simulink model "HybridBus_BackwardModel_pre_supervisory_refactor"  (R2025a)
settings: Solver=FixedStepDiscrete  StartTime=0.0  StopTime=model_stop_time_s  FixedStep=model_sample_time_s  RelTol=1e-3
InitFcn:
  | assign_hybrid_bus_model_workspace;
undefined symbols (not defined in the file or in its folder): air_density_kg_m3, auxiliary_base_power_kw, auxiliary_override, battery1_charge_efficiency, battery1_discharge_efficiency, battery1_initial_energy_kwh, battery1_max_charge_kw, battery1_max_discharge_kw, battery1_max_energy_kwh, battery1_max_soe, battery1_min_energy_kwh, battery1_usable_energy_kwh, battery2_charge_efficiency, battery2_discharge_efficiency, battery2_initial_energy_kwh, battery2_max_charge_kw, battery2_max_discharge_kw, battery2_max_energy_kwh, battery2_max_soe, battery2_min_energy_kwh, battery2_usable_energy_kwh, battery_full_detection_margin, battery_role_switch_soe, DiscIntNeverNeededParam, drag_coefficient, electricity_price_per_kWh, final_drive_motoring_efficiency, final_drive_ratio, final_drive_regen_efficiency, frontal_area_m2, fuel_price_per_L, genset_charge_target_soe, genset_fuel_L_per_kWh, genset_max_power_kw, genset_optimum_power_kw, gravity_m_s2, grid_charge_efficiency, initial_active_battery_is_1, model_sample_time_s, motor_max_speed_rpm, motor_motoring_efficiency, motor_regen_efficiency, motor_regen_limit_kw, motor_traction_limit_kw, rolling_coefficient, tyre_radius_m, vehicle_mass_kg
settings Model: Creator=Karuna  LastModifiedBy=Karuna
settings DataIOCC: SaveOutput=off  SignalLogging=off

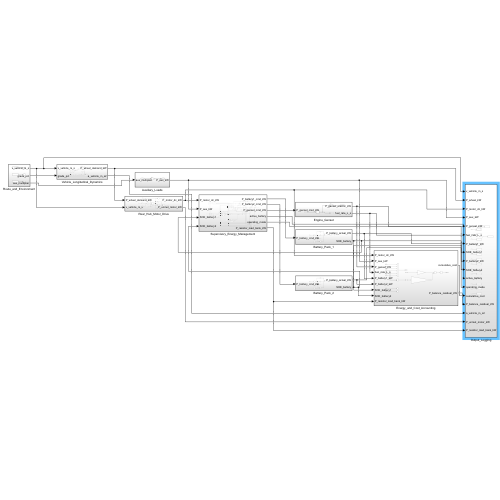
[thumbnail: Simulink's stored preview of the top-level diagram]
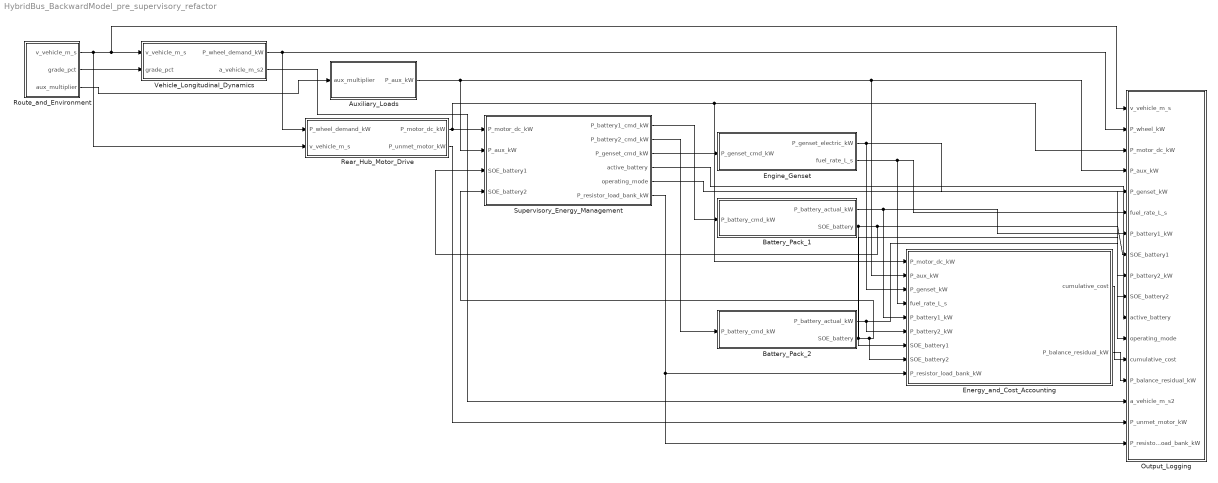
== system HybridBus_BackwardModel_pre_supervisory_refactor ==
  Auxiliary_Loads : Subsystem
  Battery_Pack_1 : Subsystem
  Battery_Pack_2 : Subsystem
  Energy_and_Cost_Accounting : Subsystem
  Engine_Genset : Subsystem
  Output_Logging : Subsystem
  Rear_Hub_Motor_Drive : Subsystem
  Route_and_Environment : Subsystem
  Supervisory_Energy_Management : Subsystem
  Vehicle_Longitudinal_Dynamics : Subsystem
  wires:
  Battery_Pack_2/2(SOE_battery) -> Supervisory_Energy_Management/4(SOE_battery2), Energy_and_Cost_Accounting/8(SOE_battery2), Output_Logging/10(SOE_battery2)
  Route_and_Environment/3(aux_multiplier) -> Auxiliary_Loads/1(aux_multiplier)
  Route_and_Environment/2(grade_pct) -> Vehicle_Longitudinal_Dynamics/2(grade_pct)
  Route_and_Environment/1(v_vehicle_m_s) -> Output_Logging/1(v_vehicle_m_s), Vehicle_Longitudinal_Dynamics/1(v_vehicle_m_s), Rear_Hub_Motor_Drive/2(v_vehicle_m_s)
  Vehicle_Longitudinal_Dynamics/1(P_wheel_demand_kW) -> Output_Logging/2(P_wheel_kW), Rear_Hub_Motor_Drive/1(P_wheel_demand_kW)
  Vehicle_Longitudinal_Dynamics/2(a_vehicle_m_s2) -> Output_Logging/15(a_vehicle_m_s2)
  Auxiliary_Loads/1(P_aux_kW) -> Energy_and_Cost_Accounting/2(P_aux_kW), Output_Logging/4(P_aux_kW), Supervisory_Energy_Management/2(P_aux_kW)
  Rear_Hub_Motor_Drive/2(P_unmet_motor_kW) -> Output_Logging/16(P_unmet_motor_kW)
  Rear_Hub_Motor_Drive/1(P_motor_dc_kW) -> Energy_and_Cost_Accounting/1(P_motor_dc_kW), Output_Logging/3(P_motor_dc_kW), Supervisory_Energy_Management/1(P_motor_dc_kW)
  Engine_Genset/2(fuel_rate_L_s) -> Energy_and_Cost_Accounting/4(fuel_rate_L_s), Output_Logging/6(fuel_rate_L_s)
  Supervisory_Energy_Management/1(P_battery1_cmd_kW) -> Battery_Pack_1/1(P_battery_cmd_kW)
  Supervisory_Energy_Management/2(P_battery2_cmd_kW) -> Battery_Pack_2/1(P_battery_cmd_kW)
  Engine_Genset/1(P_genset_electric_kW) -> Output_Logging/5(P_genset_kW), Energy_and_Cost_Accounting/3(P_genset_kW)
  Supervisory_Energy_Management/3(P_genset_cmd_kW) -> Engine_Genset/1(P_genset_cmd_kW)
  Supervisory_Energy_Management/4(active_battery) -> Output_Logging/11(active_battery)
  Supervisory_Energy_Management/5(operating_mode) -> Output_Logging/12(operating_mode)
  Supervisory_Energy_Management/6(P_resistor_load_bank_kW) -> Energy_and_Cost_Accounting/9(P_resistor_load_bank_kW), Output_Logging/17(P_resistor_load_bank_kW)
  Battery_Pack_1/1(P_battery_actual_kW) -> Output_Logging/7(P_battery1_kW), Energy_and_Cost_Accounting/5(P_battery1_kW)
  Battery_Pack_1/2(SOE_battery) -> Supervisory_Energy_Management/3(SOE_battery1), Output_Logging/8(SOE_battery1), Energy_and_Cost_Accounting/7(SOE_battery1)
  Battery_Pack_2/1(P_battery_actual_kW) -> Output_Logging/9(P_battery2_kW), Energy_and_Cost_Accounting/6(P_battery2_kW)
  Energy_and_Cost_Accounting/1(cumulative_cost) -> Output_Logging/13(cumulative_cost)
  Energy_and_Cost_Accounting/2(P_balance_residual_kW) -> Output_Logging/14(P_balance_residual_kW)

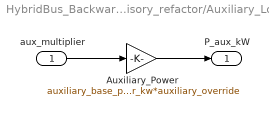
== system HybridBus_BackwardModel_pre_supervisory_refactor/Auxiliary_Loads ==
  aux_multiplier : Inport
  Auxiliary_Power : Gain  Gain=auxiliary_base_power_kw*auxiliary_override
  P_aux_kW : Outport
  wires:
  Auxiliary_Power/1 -> P_aux_kW/1
  aux_multiplier/1 -> Auxiliary_Power/1

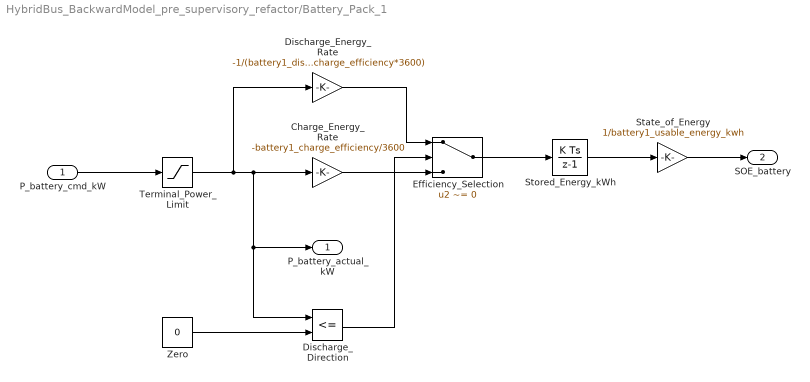
== system HybridBus_BackwardModel_pre_supervisory_refactor/Battery_Pack_1 ==
  P_battery_cmd_kW : Inport
  Charge_Energy_Rate : Gain  Gain=-battery1_charge_efficiency/3600
  Discharge_Direction : RelationalOperator  Operator=<=  OutDataTypeStr=boolean  RndMeth=Simplest  InputSameDT=off
  Discharge_Energy_Rate : Gain  Gain=-1/(battery1_discharge_efficiency*3600)
  Efficiency_Selection : Switch  Criteria=u2 ~= 0  SaturateOnIntegerOverflow=off  InputSameDT=off
  State_of_Energy : Gain  Gain=1/battery1_usable_energy_kwh
  Stored_Energy_kWh : DiscreteIntegrator  InitialCondition=battery1_initial_energy_kwh  SampleTime=model_sample_time_s  LimitOutput=on  UpperSaturationLimit=battery1_max_energy_kwh  LowerSaturationLimit=battery1_min_energy_kwh  ICPrevOutput=DiscIntNeverNeededParam  ICPrevScaledInput=DiscIntNeverNeededParam
  Terminal_Power_Limit : Saturate  UpperLimit=battery1_max_discharge_kw  LowerLimit=-battery1_max_charge_kw
  Zero : Constant  Value=0
  P_battery_actual_kW : Outport
  SOE_battery : Outport  Port=2
  wires:
  State_of_Energy/1 -> SOE_battery/1
  Stored_Energy_kWh/1 -> State_of_Energy/1
  Efficiency_Selection/1 -> Stored_Energy_kWh/1
  Charge_Energy_Rate/1 -> Efficiency_Selection/3
  Discharge_Direction/1 -> Efficiency_Selection/2
  Discharge_Energy_Rate/1 -> Efficiency_Selection/1
  Zero/1 -> Discharge_Direction/2
  Terminal_Power_Limit/1 -> P_battery_actual_kW/1, Discharge_Direction/1, Charge_Energy_Rate/1, Discharge_Energy_Rate/1
  P_battery_cmd_kW/1 -> Terminal_Power_Limit/1

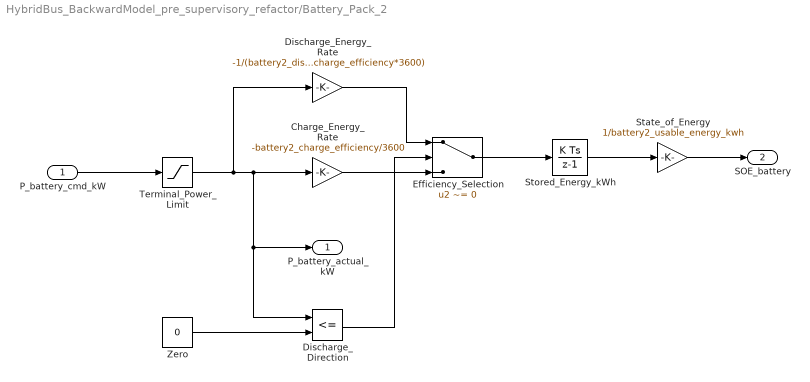
== system HybridBus_BackwardModel_pre_supervisory_refactor/Battery_Pack_2 ==
  P_battery_cmd_kW : Inport
  Charge_Energy_Rate : Gain  Gain=-battery2_charge_efficiency/3600
  Discharge_Direction : RelationalOperator  Operator=<=  OutDataTypeStr=boolean  RndMeth=Simplest  InputSameDT=off
  Discharge_Energy_Rate : Gain  Gain=-1/(battery2_discharge_efficiency*3600)
  Efficiency_Selection : Switch  Criteria=u2 ~= 0  SaturateOnIntegerOverflow=off  InputSameDT=off
  State_of_Energy : Gain  Gain=1/battery2_usable_energy_kwh
  Stored_Energy_kWh : DiscreteIntegrator  InitialCondition=battery2_initial_energy_kwh  SampleTime=model_sample_time_s  LimitOutput=on  UpperSaturationLimit=battery2_max_energy_kwh  LowerSaturationLimit=battery2_min_energy_kwh  ICPrevOutput=DiscIntNeverNeededParam  ICPrevScaledInput=DiscIntNeverNeededParam
  Terminal_Power_Limit : Saturate  UpperLimit=battery2_max_discharge_kw  LowerLimit=-battery2_max_charge_kw
  Zero : Constant  Value=0
  P_battery_actual_kW : Outport
  SOE_battery : Outport  Port=2
  wires:
  State_of_Energy/1 -> SOE_battery/1
  Stored_Energy_kWh/1 -> State_of_Energy/1
  Efficiency_Selection/1 -> Stored_Energy_kWh/1
  Charge_Energy_Rate/1 -> Efficiency_Selection/3
  Discharge_Direction/1 -> Efficiency_Selection/2
  Discharge_Energy_Rate/1 -> Efficiency_Selection/1
  Zero/1 -> Discharge_Direction/2
  Terminal_Power_Limit/1 -> P_battery_actual_kW/1, Discharge_Direction/1, Charge_Energy_Rate/1, Discharge_Energy_Rate/1
  P_battery_cmd_kW/1 -> Terminal_Power_Limit/1

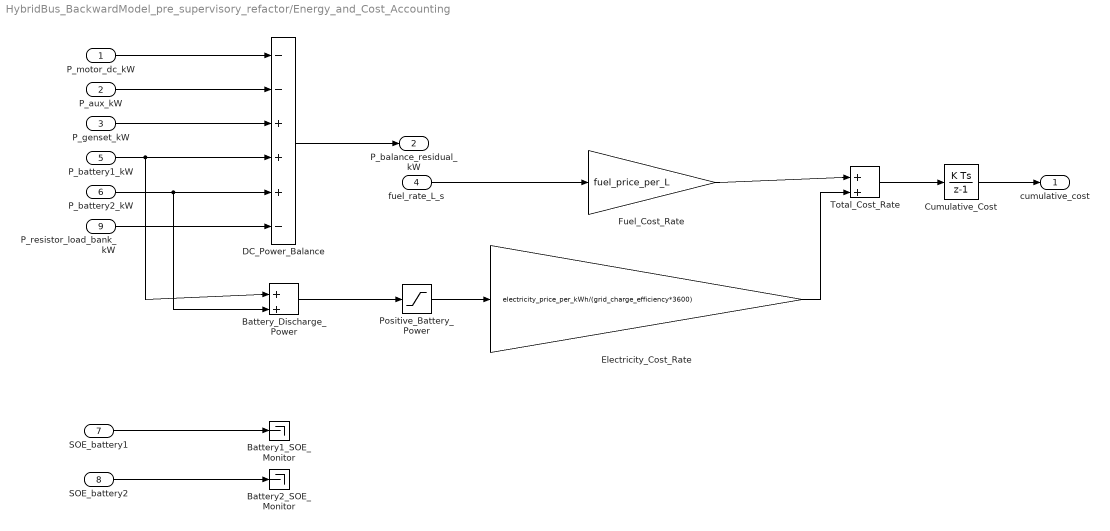
== system HybridBus_BackwardModel_pre_supervisory_refactor/Energy_and_Cost_Accounting ==
  P_motor_dc_kW : Inport
  P_aux_kW : Inport  Port=2
  P_genset_kW : Inport  Port=3
  fuel_rate_L_s : Inport  Port=4
  P_battery1_kW : Inport  Port=5
  P_battery2_kW : Inport  Port=6
  SOE_battery1 : Inport  Port=7
  SOE_battery2 : Inport  Port=8
  P_resistor_load_bank_kW : Inport  Port=9
  Battery1_SOE_Monitor : Terminator
  Battery2_SOE_Monitor : Terminator
  Battery_Discharge_Power : Sum  Inputs=|++
  Cumulative_Cost : DiscreteIntegrator  SampleTime=model_sample_time_s  ICPrevOutput=DiscIntNeverNeededParam  ICPrevScaledInput=DiscIntNeverNeededParam
  DC_Power_Balance : Sum  Inputs=--+++-
  Electricity_Cost_Rate : Gain  Gain=electricity_price_per_kWh/(grid_charge_efficiency*3600)
  Fuel_Cost_Rate : Gain  Gain=fuel_price_per_L
  Positive_Battery_Power : Saturate  UpperLimit=inf  LowerLimit=0
  Total_Cost_Rate : Sum  Inputs=|++
  cumulative_cost : Outport
  P_balance_residual_kW : Outport  Port=2
  wires:
  fuel_rate_L_s/1 -> Fuel_Cost_Rate/1
  P_aux_kW/1 -> DC_Power_Balance/2
  P_battery2_kW/1 -> Battery_Discharge_Power/2, DC_Power_Balance/5
  P_motor_dc_kW/1 -> DC_Power_Balance/1
  P_genset_kW/1 -> DC_Power_Balance/3
  P_battery1_kW/1 -> Battery_Discharge_Power/1, DC_Power_Balance/4
  SOE_battery2/1 -> Battery2_SOE_Monitor/1
  Battery_Discharge_Power/1 -> Positive_Battery_Power/1
  P_resistor_load_bank_kW/1 -> DC_Power_Balance/6
  SOE_battery1/1 -> Battery1_SOE_Monitor/1
  Cumulative_Cost/1 -> cumulative_cost/1
  DC_Power_Balance/1 -> P_balance_residual_kW/1
  Total_Cost_Rate/1 -> Cumulative_Cost/1
  Positive_Battery_Power/1 -> Electricity_Cost_Rate/1
  Fuel_Cost_Rate/1 -> Total_Cost_Rate/1
  Electricity_Cost_Rate/1 -> Total_Cost_Rate/2

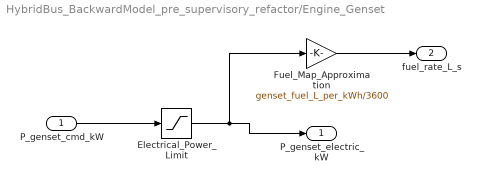
== system HybridBus_BackwardModel_pre_supervisory_refactor/Engine_Genset ==
  P_genset_cmd_kW : Inport
  Electrical_Power_Limit : Saturate  UpperLimit=genset_max_power_kw  LowerLimit=0
  Fuel_Map_Approximation : Gain  Gain=genset_fuel_L_per_kWh/3600
  P_genset_electric_kW : Outport
  fuel_rate_L_s : Outport  Port=2
  wires:
  Fuel_Map_Approximation/1 -> fuel_rate_L_s/1
  Electrical_Power_Limit/1 -> P_genset_electric_kW/1, Fuel_Map_Approximation/1
  P_genset_cmd_kW/1 -> Electrical_Power_Limit/1

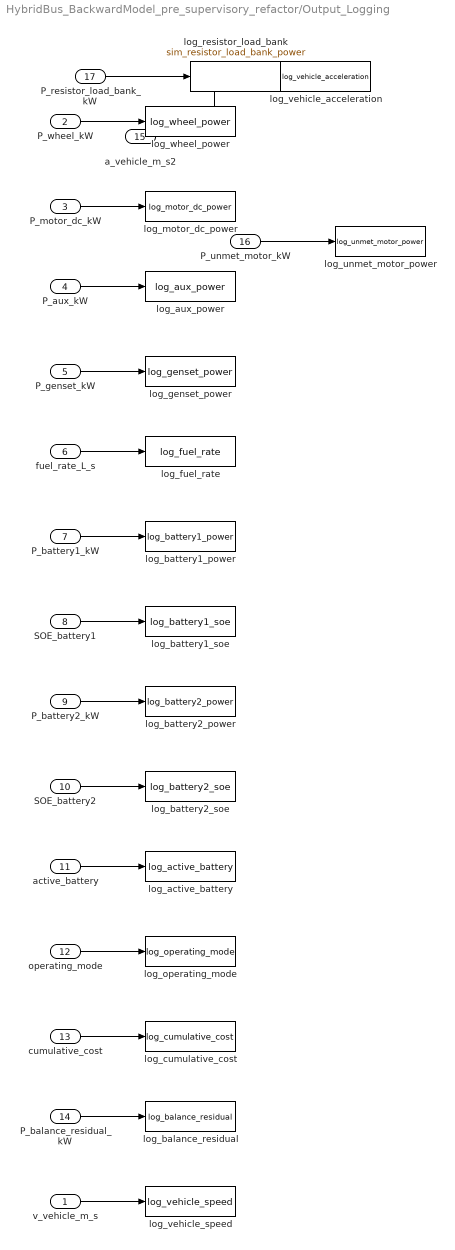
== system HybridBus_BackwardModel_pre_supervisory_refactor/Output_Logging ==
  v_vehicle_m_s : Inport
  P_wheel_kW : Inport  Port=2
  P_motor_dc_kW : Inport  Port=3
  P_aux_kW : Inport  Port=4
  P_genset_kW : Inport  Port=5
  fuel_rate_L_s : Inport  Port=6
  P_battery1_kW : Inport  Port=7
  SOE_battery1 : Inport  Port=8
  P_battery2_kW : Inport  Port=9
  SOE_battery2 : Inport  Port=10
  active_battery : Inport  Port=11
  operating_mode : Inport  Port=12
  cumulative_cost : Inport  Port=13
  P_balance_residual_kW : Inport  Port=14
  a_vehicle_m_s2 : Inport  Port=15
  P_unmet_motor_kW : Inport  Port=16
  P_resistor_load_bank_kW : Inport  Port=17
  log_active_battery : ToWorkspace  VariableName=log_active_battery  SaveFormat=Timeseries  SampleTime=-1
  log_aux_power : ToWorkspace  VariableName=log_aux_power  SaveFormat=Timeseries  SampleTime=-1
  log_balance_residual : ToWorkspace  VariableName=log_balance_residual  SaveFormat=Timeseries  SampleTime=-1
  log_battery1_power : ToWorkspace  VariableName=log_battery1_power  SaveFormat=Timeseries  SampleTime=-1
  log_battery1_soe : ToWorkspace  VariableName=log_battery1_soe  SaveFormat=Timeseries  SampleTime=-1
  log_battery2_power : ToWorkspace  VariableName=log_battery2_power  SaveFormat=Timeseries  SampleTime=-1
  log_battery2_soe : ToWorkspace  VariableName=log_battery2_soe  SaveFormat=Timeseries  SampleTime=-1
  log_cumulative_cost : ToWorkspace  VariableName=log_cumulative_cost  SaveFormat=Timeseries  SampleTime=-1
  log_fuel_rate : ToWorkspace  VariableName=log_fuel_rate  SaveFormat=Timeseries  SampleTime=-1
  log_genset_power : ToWorkspace  VariableName=log_genset_power  SaveFormat=Timeseries  SampleTime=-1
  log_motor_dc_power : ToWorkspace  VariableName=log_motor_dc_power  SaveFormat=Timeseries  SampleTime=-1
  log_operating_mode : ToWorkspace  VariableName=log_operating_mode  SaveFormat=Timeseries  SampleTime=-1
  log_resistor_load_bank : ToWorkspace  VariableName=sim_resistor_load_bank_power  SampleTime=-1
  log_unmet_motor_power : ToWorkspace  VariableName=log_unmet_motor_power  SaveFormat=Timeseries  SampleTime=-1
  log_vehicle_acceleration : ToWorkspace  VariableName=log_vehicle_acceleration  SaveFormat=Timeseries  SampleTime=-1
  log_vehicle_speed : ToWorkspace  VariableName=log_vehicle_speed  SaveFormat=Timeseries  SampleTime=-1
  log_wheel_power : ToWorkspace  VariableName=log_wheel_power  SaveFormat=Timeseries  SampleTime=-1
  wires:
  P_balance_residual_kW/1 -> log_balance_residual/1
  cumulative_cost/1 -> log_cumulative_cost/1
  operating_mode/1 -> log_operating_mode/1
  active_battery/1 -> log_active_battery/1
  SOE_battery2/1 -> log_battery2_soe/1
  P_battery2_kW/1 -> log_battery2_power/1
  SOE_battery1/1 -> log_battery1_soe/1
  P_battery1_kW/1 -> log_battery1_power/1
  fuel_rate_L_s/1 -> log_fuel_rate/1
  P_genset_kW/1 -> log_genset_power/1
  P_aux_kW/1 -> log_aux_power/1
  P_motor_dc_kW/1 -> log_motor_dc_power/1
  P_wheel_kW/1 -> log_wheel_power/1
  v_vehicle_m_s/1 -> log_vehicle_speed/1
  P_unmet_motor_kW/1 -> log_unmet_motor_power/1
  P_resistor_load_bank_kW/1 -> log_resistor_load_bank/1
  a_vehicle_m_s2/1 -> log_vehicle_acceleration/1

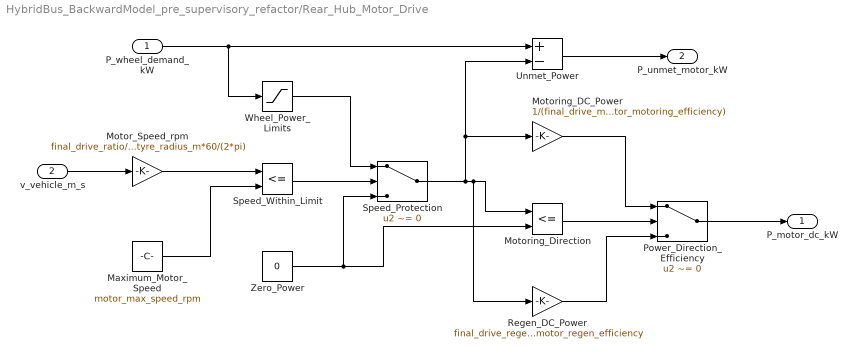
== system HybridBus_BackwardModel_pre_supervisory_refactor/Rear_Hub_Motor_Drive ==
  P_wheel_demand_kW : Inport
  v_vehicle_m_s : Inport  Port=2
  Maximum_Motor_Speed : Constant  Value=motor_max_speed_rpm
  Motor_Speed_rpm : Gain  Gain=final_drive_ratio/tyre_radius_m*60/(2*pi)
  Motoring_DC_Power : Gain  Gain=1/(final_drive_motoring_efficiency*motor_motoring_efficiency)
  Motoring_Direction : RelationalOperator  Operator=<=  OutDataTypeStr=boolean  RndMeth=Simplest  InputSameDT=off
  Power_Direction_Efficiency : Switch  Criteria=u2 ~= 0  SaturateOnIntegerOverflow=off  InputSameDT=off
  Regen_DC_Power : Gain  Gain=final_drive_regen_efficiency*motor_regen_efficiency
  Speed_Protection : Switch  Criteria=u2 ~= 0  SaturateOnIntegerOverflow=off  InputSameDT=off
  Speed_Within_Limit : RelationalOperator  Operator=<=  OutDataTypeStr=boolean  RndMeth=Simplest  InputSameDT=off
  Unmet_Power : Sum  Inputs=+-
  Wheel_Power_Limits : Saturate  UpperLimit=motor_traction_limit_kw  LowerLimit=-motor_regen_limit_kw
  Zero_Power : Constant  Value=0
  P_motor_dc_kW : Outport
  P_unmet_motor_kW : Outport  Port=2
  wires:
  Unmet_Power/1 -> P_unmet_motor_kW/1
  Power_Direction_Efficiency/1 -> P_motor_dc_kW/1
  Regen_DC_Power/1 -> Power_Direction_Efficiency/3
  Motoring_Direction/1 -> Power_Direction_Efficiency/2
  Motoring_DC_Power/1 -> Power_Direction_Efficiency/1
  Speed_Protection/1 -> Regen_DC_Power/1, Motoring_Direction/1, Motoring_DC_Power/1, Unmet_Power/2
  Zero_Power/1 -> Speed_Protection/3, Motoring_Direction/2
  Speed_Within_Limit/1 -> Speed_Protection/2
  Wheel_Power_Limits/1 -> Speed_Protection/1
  Maximum_Motor_Speed/1 -> Speed_Within_Limit/2
  Motor_Speed_rpm/1 -> Speed_Within_Limit/1
  v_vehicle_m_s/1 -> Motor_Speed_rpm/1
  P_wheel_demand_kW/1 -> Unmet_Power/1, Wheel_Power_Limits/1

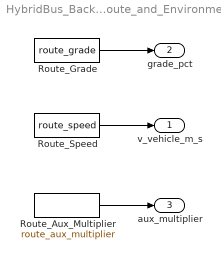
== system HybridBus_BackwardModel_pre_supervisory_refactor/Route_and_Environment ==
  Route_Aux_Multiplier : FromWorkspace  VariableName=route_aux_multiplier
  Route_Grade : FromWorkspace  VariableName=route_grade
  Route_Speed : FromWorkspace  VariableName=route_speed
  v_vehicle_m_s : Outport
  grade_pct : Outport  Port=2
  aux_multiplier : Outport  Port=3
  wires:
  Route_Aux_Multiplier/1 -> aux_multiplier/1
  Route_Grade/1 -> grade_pct/1
  Route_Speed/1 -> v_vehicle_m_s/1

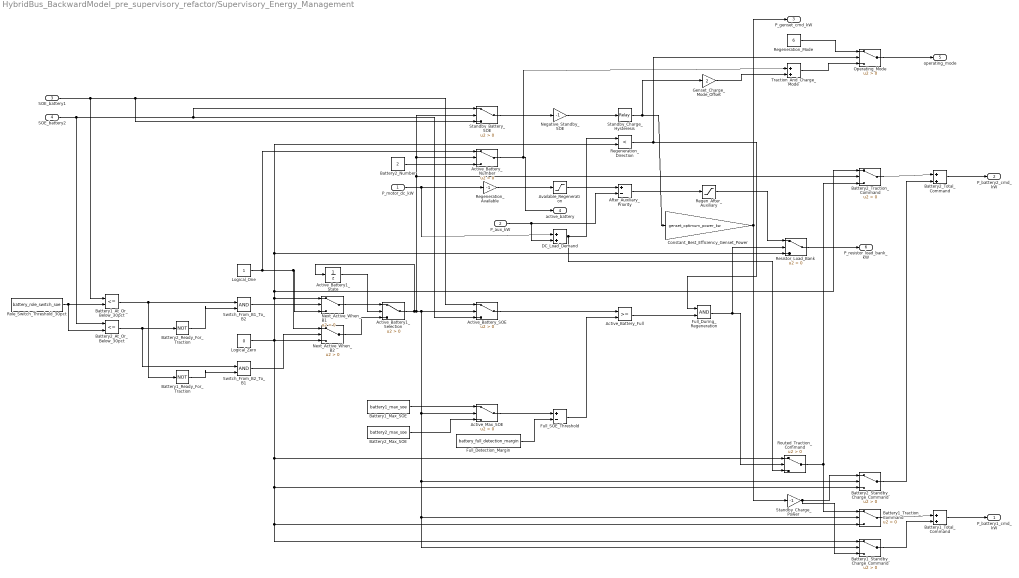
== system HybridBus_BackwardModel_pre_supervisory_refactor/Supervisory_Energy_Management ==
  P_motor_dc_kW : Inport
  P_aux_kW : Inport  Port=2
  SOE_battery1 : Inport  Port=3
  SOE_battery2 : Inport  Port=4
  Active_Battery1_Selection : Switch  Criteria=u2 > Threshold  SaturateOnIntegerOverflow=off  InputSameDT=off
  Active_Battery1_State : UnitDelay  InitialCondition=initial_active_battery_is_1  SampleTime=model_sample_time_s  HasFrameUpgradeWarning=on
  Active_Battery_Full : RelationalOperator  OutDataTypeStr=boolean  RndMeth=Simplest  InputSameDT=off
  Active_Battery_Number : Switch  Criteria=u2 > Threshold  SaturateOnIntegerOverflow=off  InputSameDT=off
  Active_Battery_SOE : Switch  Criteria=u2 > Threshold  SaturateOnIntegerOverflow=off  InputSameDT=off
  Active_Max_SOE : Switch  Criteria=u2 > Threshold  SaturateOnIntegerOverflow=off  InputSameDT=off
  After_Auxiliary_Priority : Sum  Inputs=+-
  Available_Regeneration : Saturate  UpperLimit=inf  LowerLimit=0
  Battery1_At_Or_Below_30pct : RelationalOperator  Operator=<=  OutDataTypeStr=boolean  RndMeth=Simplest  InputSameDT=off
  Battery1_Max_SOE : Constant  Value=battery1_max_soe
  Battery1_Ready_For_Traction : Logic  Operator=NOT  IconShape=distinctive  AllPortsSameDT=off  OutDataTypeStr=boolean
  Battery1_Standby_Charge_Command : Switch  Criteria=u2 > Threshold  SaturateOnIntegerOverflow=off  InputSameDT=off
  Battery1_Total_Command : Sum  Inputs=|++
  Battery1_Traction_Command : Switch  Criteria=u2 > Threshold  SaturateOnIntegerOverflow=off  InputSameDT=off
  Battery2_At_Or_Below_30pct : RelationalOperator  Operator=<=  OutDataTypeStr=boolean  RndMeth=Simplest  InputSameDT=off
  Battery2_Max_SOE : Constant  Value=battery2_max_soe
  Battery2_Number : Constant  Value=2
  Battery2_Ready_For_Traction : Logic  Operator=NOT  IconShape=distinctive  AllPortsSameDT=off  OutDataTypeStr=boolean
  Battery2_Standby_Charge_Command : Switch  Criteria=u2 > Threshold  SaturateOnIntegerOverflow=off  InputSameDT=off
  Battery2_Total_Command : Sum  Inputs=|++
  Battery2_Traction_Command : Switch  Criteria=u2 > Threshold  SaturateOnIntegerOverflow=off  InputSameDT=off
  Constant_Best_Efficiency_Genset_Power : Gain  Gain=genset_optimum_power_kw
  DC_Load_Demand : Sum  Inputs=|++
  Full_Detection_Margin : Constant  Value=battery_full_detection_margin
  Full_During_Regeneration : Logic  AllPortsSameDT=off  OutDataTypeStr=boolean
  Full_SOE_Threshold : Sum  Inputs=+-
  Genset_Charge_Mode_Offset : Gain  Gain=2
  Logical_One : Constant
  Logical_Zero : Constant  Value=0
  Negative_Standby_SOE : Gain  Gain=-1
  Next_Active_When_B1 : Switch  Criteria=u2 > Threshold  SaturateOnIntegerOverflow=off  InputSameDT=off
  Next_Active_When_B2 : Switch  Criteria=u2 > Threshold  SaturateOnIntegerOverflow=off  InputSameDT=off
  Operating_Mode : Switch  Criteria=u2 > Threshold  SaturateOnIntegerOverflow=off  InputSameDT=off
  Regen_After_Auxiliary : Saturate  UpperLimit=inf  LowerLimit=0
  Regeneration_Available : Gain  Gain=-1
  Regeneration_Direction : RelationalOperator  Operator=<  OutDataTypeStr=boolean  RndMeth=Simplest  InputSameDT=off
  Regeneration_Mode : Constant  Value=6
  Resistor_Load_Bank : Switch  Criteria=u2 > Threshold  SaturateOnIntegerOverflow=off  InputSameDT=off
  Role_Switch_Threshold_30pct : Constant  Value=battery_role_switch_soe
  Routed_Traction_Command : Switch  Criteria=u2 > Threshold  SaturateOnIntegerOverflow=off  InputSameDT=off
  Standby_Battery_SOE : Switch  Criteria=u2 > Threshold  SaturateOnIntegerOverflow=off  InputSameDT=off
  Standby_Charge_Hysteresis : Relay  OnSwitchValue=-battery_role_switch_soe  OffSwitchValue=-genset_charge_target_soe
  Standby_Charge_Power : Gain  Gain=-1
  Switch_From_B1_To_B2 : Logic  IconShape=distinctive  AllPortsSameDT=off  OutDataTypeStr=boolean
  Switch_From_B2_To_B1 : Logic  IconShape=distinctive  AllPortsSameDT=off  OutDataTypeStr=boolean
  Traction_And_Charge_Mode : Sum  Inputs=|++
  P_battery1_cmd_kW : Outport
  P_battery2_cmd_kW : Outport  Port=2
  P_genset_cmd_kW : Outport  Port=3
  active_battery : Outport  Port=4
  operating_mode : Outport  Port=5
  P_resistor_load_bank_kW : Outport  Port=6
  wires:
  Active_Battery1_State/1 -> Active_Battery1_Selection/2
  SOE_battery2/1 -> Active_Battery_SOE/3, Standby_Battery_SOE/1, Battery2_At_Or_Below_30pct/1
  SOE_battery1/1 -> Active_Battery_SOE/1, Standby_Battery_SOE/3, Battery1_At_Or_Below_30pct/1
  Regen_After_Auxiliary/1 -> Resistor_Load_Bank/1
  Next_Active_When_B2/1 -> Active_Battery1_Selection/3
  Role_Switch_Threshold_30pct/1 -> Battery2_At_Or_Below_30pct/2, Battery1_At_Or_Below_30pct/2
  Battery1_Ready_For_Traction/1 -> Switch_From_B2_To_B1/2
  Active_Battery_SOE/1 -> Active_Battery_Full/1
  Battery1_At_Or_Below_30pct/1 -> Battery1_Ready_For_Traction/1, Switch_From_B1_To_B2/1
  Battery2_Total_Command/1 -> P_battery2_cmd_kW/1
  Battery2_At_Or_Below_30pct/1 -> Switch_From_B2_To_B1/1, Battery2_Ready_For_Traction/1
  Battery2_Ready_For_Traction/1 -> Switch_From_B1_To_B2/2
  Logical_One/1 -> Next_Active_When_B1/3, Next_Active_When_B2/1, Active_Battery_Number/1
  Traction_And_Charge_Mode/1 -> Operating_Mode/3
  Switch_From_B1_To_B2/1 -> Next_Active_When_B1/2
  Battery2_Traction_Command/1 -> Battery2_Total_Command/1
  Logical_Zero/1 -> Battery1_Traction_Command/3, Battery1_Standby_Charge_Command/1, Battery2_Standby_Charge_Command/3, Routed_Traction_Command/1, Resistor_Load_Bank/3, Regeneration_Direction/2, Battery2_Traction_Command/1, Next_Active_When_B1/1, Next_Active_When_B2/3
  Standby_Charge_Power/1 -> Battery1_Standby_Charge_Command/3, Battery2_Standby_Charge_Command/1
  Switch_From_B2_To_B1/1 -> Next_Active_When_B2/2
  Regeneration_Available/1 -> Available_Regeneration/1
  Next_Active_When_B1/1 -> Active_Battery1_Selection/1
  Battery1_Traction_Command/1 -> Battery1_Total_Command/1
  Battery2_Standby_Charge_Command/1 -> Battery2_Total_Command/2
  Battery2_Number/1 -> Active_Battery_Number/3
  P_motor_dc_kW/1 -> DC_Load_Demand/1, Regeneration_Available/1
  Active_Battery1_Selection/1 -> Battery1_Traction_Command/2, Battery1_Standby_Charge_Command/2, Battery2_Standby_Charge_Command/2, Active_Max_SOE/2, Active_Battery_SOE/2, Standby_Battery_SOE/2, Active_Battery_Number/2, Battery2_Traction_Command/2, Active_Battery1_State/1
  Battery1_Max_SOE/1 -> Active_Max_SOE/1
  Battery2_Max_SOE/1 -> Active_Max_SOE/3
  Standby_Battery_SOE/1 -> Negative_Standby_SOE/1
  Active_Battery_Number/1 -> Traction_And_Charge_Mode/1, active_battery/1
  Active_Battery_Full/1 -> Full_During_Regeneration/2
  P_aux_kW/1 -> After_Auxiliary_Priority/2, DC_Load_Demand/2
  Active_Max_SOE/1 -> Full_SOE_Threshold/1
  Full_SOE_Threshold/1 -> Active_Battery_Full/2
  Full_Detection_Margin/1 -> Full_SOE_Threshold/2
  Constant_Best_Efficiency_Genset_Power/1 -> P_genset_cmd_kW/1, Standby_Charge_Power/1
  Negative_Standby_SOE/1 -> Standby_Charge_Hysteresis/1
  Available_Regeneration/1 -> After_Auxiliary_Priority/1
  DC_Load_Demand/1 -> Routed_Traction_Command/3, Regeneration_Direction/1
  Routed_Traction_Command/1 -> Battery2_Traction_Command/3, Battery1_Traction_Command/1
  Standby_Charge_Hysteresis/1 -> Constant_Best_Efficiency_Genset_Power/1, Genset_Charge_Mode_Offset/1
  Regeneration_Direction/1 -> Full_During_Regeneration/1, Operating_Mode/2
  After_Auxiliary_Priority/1 -> Regen_After_Auxiliary/1
  Genset_Charge_Mode_Offset/1 -> Traction_And_Charge_Mode/2
  Full_During_Regeneration/1 -> Routed_Traction_Command/2, Resistor_Load_Bank/2
  Regeneration_Mode/1 -> Operating_Mode/1
  Resistor_Load_Bank/1 -> P_resistor_load_bank_kW/1
  Operating_Mode/1 -> operating_mode/1
  Battery1_Standby_Charge_Command/1 -> Battery1_Total_Command/2
  Battery1_Total_Command/1 -> P_battery1_cmd_kW/1

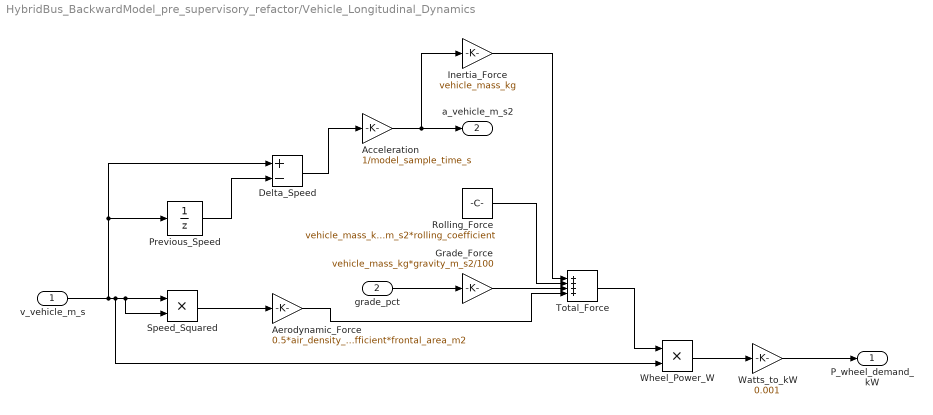
== system HybridBus_BackwardModel_pre_supervisory_refactor/Vehicle_Longitudinal_Dynamics ==
  v_vehicle_m_s : Inport
  grade_pct : Inport  Port=2
  Acceleration : Gain  Gain=1/model_sample_time_s
  Aerodynamic_Force : Gain  Gain=0.5*air_density_kg_m3*drag_coefficient*frontal_area_m2
  Delta_Speed : Sum  Inputs=+-
  Grade_Force : Gain  Gain=vehicle_mass_kg*gravity_m_s2/100
  Inertia_Force : Gain  Gain=vehicle_mass_kg
  Previous_Speed : UnitDelay  SampleTime=model_sample_time_s  HasFrameUpgradeWarning=on
  Rolling_Force : Constant  Value=vehicle_mass_kg*gravity_m_s2*rolling_coefficient
  Speed_Squared : Product  Inputs=**
  Total_Force : Sum  Inputs=++++
  Watts_to_kW : Gain  Gain=0.001
  Wheel_Power_W : Product  Inputs=**
  P_wheel_demand_kW : Outport
  a_vehicle_m_s2 : Outport  Port=2
  wires:
  Watts_to_kW/1 -> P_wheel_demand_kW/1
  Wheel_Power_W/1 -> Watts_to_kW/1
  Total_Force/1 -> Wheel_Power_W/1
  Aerodynamic_Force/1 -> Total_Force/4
  Grade_Force/1 -> Total_Force/3
  Rolling_Force/1 -> Total_Force/2
  Inertia_Force/1 -> Total_Force/1
  Speed_Squared/1 -> Aerodynamic_Force/1
  grade_pct/1 -> Grade_Force/1
  Acceleration/1 -> a_vehicle_m_s2/1, Inertia_Force/1
  Delta_Speed/1 -> Acceleration/1
  Previous_Speed/1 -> Delta_Speed/2
  v_vehicle_m_s/1 -> Speed_Squared/1, Speed_Squared/2, Wheel_Power_W/2, Previous_Speed/1, Delta_Speed/1
